simulink model "path_following_revised"  (R2016a)
settings: Solver=ode4  StartTime=0.0  StopTime=2000  FixedStep=0.001  MaxStep=0.01  RelTol=1e-6
values from neighbouring files (symbols this model uses):
  float =     [waveglider.mat]
  floatABC =     [waveglider.mat]
  gliderABC =     [waveglider.mat]
undefined symbols (not defined in the file or in its folder): magnitude, RAO_Vel
libraries: simulink_extras x8, simulink x5, marine_gnc x4, fuzblock x1, marine_hydro x1
(part 3 of 3)

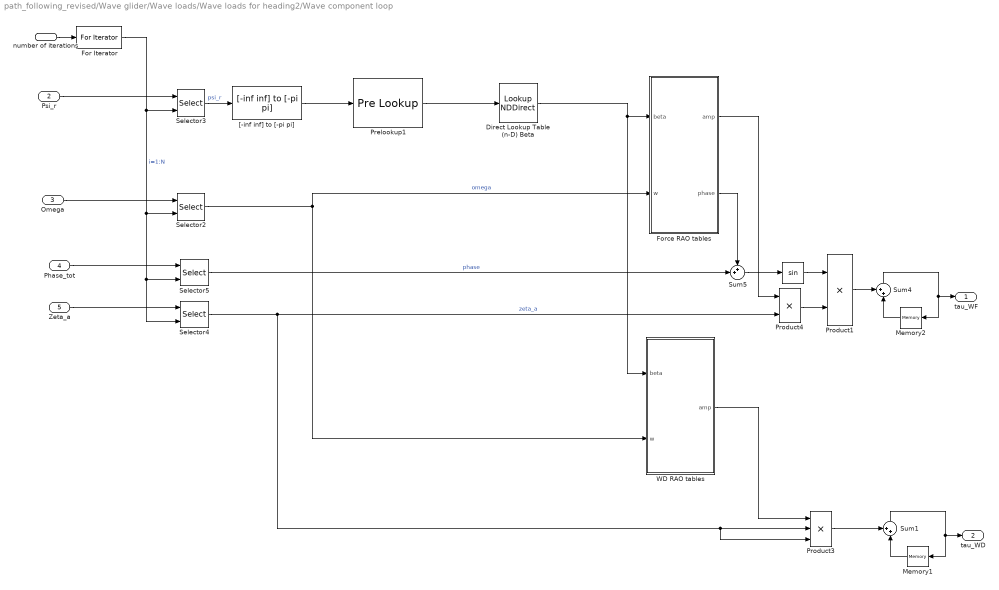
== system path_following_revised/Wave glider/Wave loads/Wave loads for heading2/Wave component loop ==
  number of iterations : Inport
  Psi_r : Inport  Port=2
  Omega : Inport  Port=3
  Phase_tot : Inport  Port=4
  Zeta_a : Inport  Port=5
  "                " : Trigonometry
  Direct Lookup Table (n-D) Beta : LookupNDDirect  NumberOfTableDimensions=1  Table=float.headings
  For Iterator : ForIterator  ResetStates=reset  IterationSource=external  IterationVariableDataType=double
  Force RAO tables : Subsystem  mask(RAO table lookup){}
      mask help:
      | Perform 3D table lookup in 6DOF RAO amplitudes and phases, using the relative wave heading psi_r, wave frequency omega and vessel velocity vel as inputs. See documentation of the Motion RAO block or Force RAO block for details. A warning is issued if the input is outside the range spanned by the RAOs.
      |
      | Author: Oyvind N. Smogeli and Thor I. Fossen, 2005-05-03
  Memory1 : Memory  X0=[0 0 0 0 0 0]'  InheritSampleTime=on
  Memory2 : Memory  X0=[0 0 0 0 0 0]'  InheritSampleTime=on
  Prelookup1 : PreLookup  BreakpointsData=float.headings  IndexSearchMethod=Linear search  BeginIndexSearchUsingPreviousIndexResult=on  OutputOnlyTheIndex=on
  Product1 : Product  SaturateOnIntegerOverflow=on  OutDataTypeStr=Inherit: Same as first input
  Product3 : Product  Inputs=3  SaturateOnIntegerOverflow=on  OutDataTypeStr=Inherit: Same as first input
  Product4 : Product  SaturateOnIntegerOverflow=on  OutDataTypeStr=Inherit: Same as first input
  Selector{2..5} (4 alike) : Selector  IndexOptions=Index vector (port)  Indices=[1 3]  OutputSizes=1
  Sum1 : Sum  Inputs=++|  SaturateOnIntegerOverflow=on
  Sum4 : Sum  Inputs=++|  SaturateOnIntegerOverflow=on
  Sum5 : Sum  Inputs=++|  SaturateOnIntegerOverflow=on
  WD RAO tables : Subsystem  mask(RAO table lookup){}
      mask help:
      | Perform 3D table lookup in 6DOF RAO amplitudes and phases, using the relative wave heading psi_r, wave frequency omega and vessel velocity vel as inputs. See documentation of the Motion RAO block or Force RAO block for details. A warning is issued if the input is outside the range spanned by the RAOs.
      |
      | Author: Oyvind N. Smogeli and Thor I. Fossen, 2005-05-03
  "[-inf inf] to [-pi pi]" : marine_gnc/Utilities/Math Operations/[-inf inf] to [-pi pi]
  tau_WF : Outport
  tau_WD : Outport  Port=2
  wires:
  WD RAO tables/1(amp) -> Product3/1
  Force RAO tables/1(amp) -> Product4/1
  Force RAO tables/2(phase) -> Sum5/1
  Direct Lookup Table (n-D) Beta/1 -> WD RAO tables/1(beta), Force RAO tables/1(beta)
  Prelookup1/1 -> Direct Lookup Table (n-D) Beta/1
  For Iterator/1 -> Selector5/2, Selector4/2, Selector2/2, Selector3/2  "i=1:N"
  Selector2/1 -> WD RAO tables/2(w), Force RAO tables/2(w)  "omega"
  "[-inf inf] to [-pi pi]"/1 -> Prelookup1/1
  Product3/1 -> Sum1/1
  Memory1/1 -> Sum1/2
  Sum1/1 -> tau_WD/1, Memory1/1
  Product4/1 -> Product1/2
  "                "/1 -> Product1/1
  Selector3/1 -> "[-inf inf] to [-pi pi]"/1  "psi_r"
  Selector5/1 -> Sum5/2  "phase"
  Product1/1 -> Sum4/1
  Memory2/1 -> Sum4/2
  Sum4/1 -> tau_WF/1, Memory2/1
  number of iterations/1 -> For Iterator/1
  Omega/1 -> Selector2/1
  Psi_r/1 -> Selector3/1
  Phase_tot/1 -> Selector5/1
  Zeta_a/1 -> Selector4/1
  Sum5/1 -> "                "/1
  Selector4/1 -> Product3/3, Product3/2, Product4/2  "zeta_a"

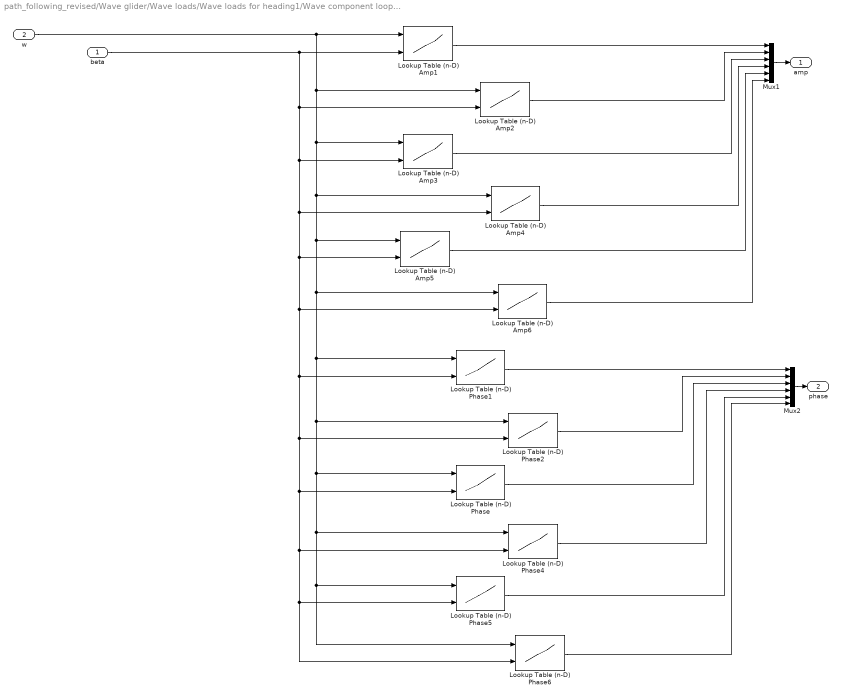
== system path_following_revised/Wave glider/Wave loads/Wave loads for heading1/Wave component loop/Force RAO tables ==
  beta : Inport
  w : Inport  Port=2
  Lookup Table (n-D) Amp1 : Lookup_n-D  BreakpointsForDimension1=float.forceRAO.w  BreakpointsForDimension2=float.headings  BreakpointsForDimension3=RAO_Vel  IndexSearchMethod=Linear search  BeginIndexSearchUsingPreviousIndexResult=on  Table=float.forceRAO.amp{1}  ExtrapMethod=Clip  DiagnosticForOutOfRangeInput=Warning  InternalRulePriority=Speed  RndMeth=Simplest  InputSameDT=on
  Lookup Table (n-D) Amp2 : Lookup_n-D  BreakpointsForDimension1=float.forceRAO.w  BreakpointsForDimension2=float.headings  BreakpointsForDimension3=RAO_Vel  IndexSearchMethod=Linear search  BeginIndexSearchUsingPreviousIndexResult=on  Table=float.forceRAO.amp{2}  ExtrapMethod=Clip  DiagnosticForOutOfRangeInput=Warning  InternalRulePriority=Speed  RndMeth=Simplest  InputSameDT=on
  Lookup Table (n-D) Amp3 : Lookup_n-D  BreakpointsForDimension1=float.forceRAO.w  BreakpointsForDimension2=float.headings  BreakpointsForDimension3=RAO_Vel  IndexSearchMethod=Linear search  BeginIndexSearchUsingPreviousIndexResult=on  Table=float.forceRAO.amp{3}  ExtrapMethod=Clip  DiagnosticForOutOfRangeInput=Warning  InternalRulePriority=Speed  RndMeth=Simplest  InputSameDT=on
  Lookup Table (n-D) Amp4 : Lookup_n-D  BreakpointsForDimension1=float.forceRAO.w  BreakpointsForDimension2=float.headings  BreakpointsForDimension3=RAO_Vel  IndexSearchMethod=Linear search  BeginIndexSearchUsingPreviousIndexResult=on  Table=float.forceRAO.amp{4}  ExtrapMethod=Clip  DiagnosticForOutOfRangeInput=Warning  InternalRulePriority=Speed  RndMeth=Simplest  InputSameDT=on
  Lookup Table (n-D) Amp5 : Lookup_n-D  BreakpointsForDimension1=float.forceRAO.w  BreakpointsForDimension2=float.headings  BreakpointsForDimension3=RAO_Vel  IndexSearchMethod=Linear search  BeginIndexSearchUsingPreviousIndexResult=on  Table=float.forceRAO.amp{5}  ExtrapMethod=Clip  DiagnosticForOutOfRangeInput=Warning  InternalRulePriority=Speed  RndMeth=Simplest  InputSameDT=on
  Lookup Table (n-D) Amp6 : Lookup_n-D  BreakpointsForDimension1=float.forceRAO.w  BreakpointsForDimension2=float.headings  BreakpointsForDimension3=RAO_Vel  IndexSearchMethod=Linear search  BeginIndexSearchUsingPreviousIndexResult=on  Table=float.forceRAO.amp{6}  ExtrapMethod=Clip  DiagnosticForOutOfRangeInput=Warning  InternalRulePriority=Speed  RndMeth=Simplest  InputSameDT=on
  Lookup Table (n-D) Phase : Lookup_n-D  BreakpointsForDimension1=float.forceRAO.w  BreakpointsForDimension2=float.headings  BreakpointsForDimension3=RAO_Vel  IndexSearchMethod=Linear search  BeginIndexSearchUsingPreviousIndexResult=on  Table=float.forceRAO.phase{3}  ExtrapMethod=Clip  DiagnosticForOutOfRangeInput=Warning  InternalRulePriority=Speed  RndMeth=Simplest  InputSameDT=on
  Lookup Table (n-D) Phase1 : Lookup_n-D  BreakpointsForDimension1=float.forceRAO.w  BreakpointsForDimension2=float.headings  BreakpointsForDimension3=RAO_Vel  IndexSearchMethod=Linear search  BeginIndexSearchUsingPreviousIndexResult=on  Table=float.forceRAO.phase{1}  ExtrapMethod=Clip  DiagnosticForOutOfRangeInput=Warning  InternalRulePriority=Speed  RndMeth=Simplest  InputSameDT=on
  Lookup Table (n-D) Phase2 : Lookup_n-D  BreakpointsForDimension1=float.forceRAO.w  BreakpointsForDimension2=float.headings  BreakpointsForDimension3=RAO_Vel  IndexSearchMethod=Linear search  BeginIndexSearchUsingPreviousIndexResult=on  Table=float.forceRAO.phase{2}  ExtrapMethod=Clip  DiagnosticForOutOfRangeInput=Warning  InternalRulePriority=Speed  RndMeth=Simplest  InputSameDT=on
  Lookup Table (n-D) Phase4 : Lookup_n-D  BreakpointsForDimension1=float.forceRAO.w  BreakpointsForDimension2=float.headings  BreakpointsForDimension3=RAO_Vel  IndexSearchMethod=Linear search  BeginIndexSearchUsingPreviousIndexResult=on  Table=float.forceRAO.phase{4}  ExtrapMethod=Clip  DiagnosticForOutOfRangeInput=Warning  InternalRulePriority=Speed  RndMeth=Simplest  InputSameDT=on
  Lookup Table (n-D) Phase5 : Lookup_n-D  BreakpointsForDimension1=float.forceRAO.w  BreakpointsForDimension2=float.headings  BreakpointsForDimension3=RAO_Vel  IndexSearchMethod=Linear search  BeginIndexSearchUsingPreviousIndexResult=on  Table=float.forceRAO.phase{5}  ExtrapMethod=Clip  DiagnosticForOutOfRangeInput=Warning  InternalRulePriority=Speed  RndMeth=Simplest  InputSameDT=on
  Lookup Table (n-D) Phase6 : Lookup_n-D  BreakpointsForDimension1=float.forceRAO.w  BreakpointsForDimension2=float.headings  BreakpointsForDimension3=RAO_Vel  IndexSearchMethod=Linear search  BeginIndexSearchUsingPreviousIndexResult=on  Table=float.forceRAO.phase{6}  ExtrapMethod=Clip  DiagnosticForOutOfRangeInput=Warning  InternalRulePriority=Speed  RndMeth=Simplest  InputSameDT=on
  Mux1 : Mux  Inputs=6
  Mux2 : Mux  Inputs=6
  amp : Outport
  phase : Outport  Port=2
  wires:
  w/1 -> Lookup Table (n-D) Amp1/1, Lookup Table (n-D) Amp2/1, Lookup Table (n-D) Amp3/1, Lookup Table (n-D) Amp4/1, Lookup Table (n-D) Amp5/1, Lookup Table (n-D) Amp6/1, Lookup Table (n-D) Phase1/1, Lookup Table (n-D) Phase2/1, Lookup Table (n-D) Phase/1, Lookup Table (n-D) Phase4/1, Lookup Table (n-D) Phase6/1, Lookup Table (n-D) Phase5/1
  Lookup Table (n-D) Phase5/1 -> Mux2/5
  Lookup Table (n-D) Phase/1 -> Mux2/3
  Lookup Table (n-D) Phase1/1 -> Mux2/1
  beta/1 -> Lookup Table (n-D) Amp1/2, Lookup Table (n-D) Amp2/2, Lookup Table (n-D) Amp3/2, Lookup Table (n-D) Amp4/2, Lookup Table (n-D) Amp6/2, Lookup Table (n-D) Phase1/2, Lookup Table (n-D) Phase2/2, Lookup Table (n-D) Phase/2, Lookup Table (n-D) Phase4/2, Lookup Table (n-D) Phase6/2, Lookup Table (n-D) Phase5/2, Lookup Table (n-D) Amp5/2
  Lookup Table (n-D) Phase4/1 -> Mux2/4
  Lookup Table (n-D) Phase2/1 -> Mux2/2
  Lookup Table (n-D) Phase6/1 -> Mux2/6
  Lookup Table (n-D) Amp4/1 -> Mux1/4
  Lookup Table (n-D) Amp1/1 -> Mux1/1
  Lookup Table (n-D) Amp3/1 -> Mux1/3
  Lookup Table (n-D) Amp5/1 -> Mux1/5
  Lookup Table (n-D) Amp2/1 -> Mux1/2
  Lookup Table (n-D) Amp6/1 -> Mux1/6
  Mux2/1 -> phase/1
  Mux1/1 -> amp/1

== system path_following_revised/Wave glider/Wave loads/Wave loads for heading1/Wave component loop/WD RAO tables ==
  beta : Inport
  w : Inport  Port=2
  Constant : Constant  Value=0
  Lookup Table (n-D) Wavedrift 1 : Lookup_n-D  BreakpointsForDimension1=float.driftfrc.w  BreakpointsForDimension2=float.headings  BreakpointsForDimension3=RAO_Vel  IndexSearchMethod=Linear search  BeginIndexSearchUsingPreviousIndexResult=on  Table=float.driftfrc.amp{1}  ExtrapMethod=Clip  DiagnosticForOutOfRangeInput=Warning  InternalRulePriority=Speed  RndMeth=Simplest  InputSameDT=on
  Lookup Table (n-D) Wavedrift 2 : Lookup_n-D  BreakpointsForDimension1=float.driftfrc.w  BreakpointsForDimension2=float.headings  BreakpointsForDimension3=RAO_Vel  IndexSearchMethod=Linear search  BeginIndexSearchUsingPreviousIndexResult=on  Table=float.driftfrc.amp{2}  ExtrapMethod=Clip  DiagnosticForOutOfRangeInput=Warning  InternalRulePriority=Speed  RndMeth=Simplest  InputSameDT=on
  Lookup Table (n-D) Wavedrift 3 : Lookup_n-D  BreakpointsForDimension1=float.driftfrc.w  BreakpointsForDimension2=float.headings  BreakpointsForDimension3=RAO_Vel  IndexSearchMethod=Linear search  BeginIndexSearchUsingPreviousIndexResult=on  Table=float.driftfrc.amp{3}  ExtrapMethod=Clip  DiagnosticForOutOfRangeInput=Warning  InternalRulePriority=Speed  RndMeth=Simplest  InputSameDT=on
  Mux1 : Mux  Inputs=6
  amp : Outport
  wires:
  w/1 -> Lookup Table (n-D) Wavedrift 1/1, Lookup Table (n-D) Wavedrift 3/1, Lookup Table (n-D) Wavedrift 2/1
  Constant/1 -> Mux1/5, Mux1/4, Mux1/3
  beta/1 -> Lookup Table (n-D) Wavedrift 1/2, Lookup Table (n-D) Wavedrift 3/2, Lookup Table (n-D) Wavedrift 2/2
  Lookup Table (n-D) Wavedrift 1/1 -> Mux1/1
  Lookup Table (n-D) Wavedrift 2/1 -> Mux1/2
  Lookup Table (n-D) Wavedrift 3/1 -> Mux1/6
  Mux1/1 -> amp/1

== system path_following_revised/Wave glider/Wave loads/Wave loads for heading2/Wave component loop/Force RAO tables ==
  beta : Inport
  w : Inport  Port=2
  Lookup Table (n-D) Amp1 : Lookup_n-D  BreakpointsForDimension1=float.forceRAO.w  BreakpointsForDimension2=float.headings  BreakpointsForDimension3=RAO_Vel  IndexSearchMethod=Linear search  BeginIndexSearchUsingPreviousIndexResult=on  Table=float.forceRAO.amp{1}  ExtrapMethod=Clip  DiagnosticForOutOfRangeInput=Warning  InternalRulePriority=Speed  RndMeth=Simplest  InputSameDT=on
  Lookup Table (n-D) Amp2 : Lookup_n-D  BreakpointsForDimension1=float.forceRAO.w  BreakpointsForDimension2=float.headings  BreakpointsForDimension3=RAO_Vel  IndexSearchMethod=Linear search  BeginIndexSearchUsingPreviousIndexResult=on  Table=float.forceRAO.amp{2}  ExtrapMethod=Clip  DiagnosticForOutOfRangeInput=Warning  InternalRulePriority=Speed  RndMeth=Simplest  InputSameDT=on
  Lookup Table (n-D) Amp3 : Lookup_n-D  BreakpointsForDimension1=float.forceRAO.w  BreakpointsForDimension2=float.headings  BreakpointsForDimension3=RAO_Vel  IndexSearchMethod=Linear search  BeginIndexSearchUsingPreviousIndexResult=on  Table=float.forceRAO.amp{3}  ExtrapMethod=Clip  DiagnosticForOutOfRangeInput=Warning  InternalRulePriority=Speed  RndMeth=Simplest  InputSameDT=on
  Lookup Table (n-D) Amp4 : Lookup_n-D  BreakpointsForDimension1=float.forceRAO.w  BreakpointsForDimension2=float.headings  BreakpointsForDimension3=RAO_Vel  IndexSearchMethod=Linear search  BeginIndexSearchUsingPreviousIndexResult=on  Table=float.forceRAO.amp{4}  ExtrapMethod=Clip  DiagnosticForOutOfRangeInput=Warning  InternalRulePriority=Speed  RndMeth=Simplest  InputSameDT=on
  Lookup Table (n-D) Amp5 : Lookup_n-D  BreakpointsForDimension1=float.forceRAO.w  BreakpointsForDimension2=float.headings  BreakpointsForDimension3=RAO_Vel  IndexSearchMethod=Linear search  BeginIndexSearchUsingPreviousIndexResult=on  Table=float.forceRAO.amp{5}  ExtrapMethod=Clip  DiagnosticForOutOfRangeInput=Warning  InternalRulePriority=Speed  RndMeth=Simplest  InputSameDT=on
  Lookup Table (n-D) Amp6 : Lookup_n-D  BreakpointsForDimension1=float.forceRAO.w  BreakpointsForDimension2=float.headings  BreakpointsForDimension3=RAO_Vel  IndexSearchMethod=Linear search  BeginIndexSearchUsingPreviousIndexResult=on  Table=float.forceRAO.amp{6}  ExtrapMethod=Clip  DiagnosticForOutOfRangeInput=Warning  InternalRulePriority=Speed  RndMeth=Simplest  InputSameDT=on
  Lookup Table (n-D) Phase : Lookup_n-D  BreakpointsForDimension1=float.forceRAO.w  BreakpointsForDimension2=float.headings  BreakpointsForDimension3=RAO_Vel  IndexSearchMethod=Linear search  BeginIndexSearchUsingPreviousIndexResult=on  Table=float.forceRAO.phase{3}  ExtrapMethod=Clip  DiagnosticForOutOfRangeInput=Warning  InternalRulePriority=Speed  RndMeth=Simplest  InputSameDT=on
  Lookup Table (n-D) Phase1 : Lookup_n-D  BreakpointsForDimension1=float.forceRAO.w  BreakpointsForDimension2=float.headings  BreakpointsForDimension3=RAO_Vel  IndexSearchMethod=Linear search  BeginIndexSearchUsingPreviousIndexResult=on  Table=float.forceRAO.phase{1}  ExtrapMethod=Clip  DiagnosticForOutOfRangeInput=Warning  InternalRulePriority=Speed  RndMeth=Simplest  InputSameDT=on
  Lookup Table (n-D) Phase2 : Lookup_n-D  BreakpointsForDimension1=float.forceRAO.w  BreakpointsForDimension2=float.headings  BreakpointsForDimension3=RAO_Vel  IndexSearchMethod=Linear search  BeginIndexSearchUsingPreviousIndexResult=on  Table=float.forceRAO.phase{2}  ExtrapMethod=Clip  DiagnosticForOutOfRangeInput=Warning  InternalRulePriority=Speed  RndMeth=Simplest  InputSameDT=on
  Lookup Table (n-D) Phase4 : Lookup_n-D  BreakpointsForDimension1=float.forceRAO.w  BreakpointsForDimension2=float.headings  BreakpointsForDimension3=RAO_Vel  IndexSearchMethod=Linear search  BeginIndexSearchUsingPreviousIndexResult=on  Table=float.forceRAO.phase{4}  ExtrapMethod=Clip  DiagnosticForOutOfRangeInput=Warning  InternalRulePriority=Speed  RndMeth=Simplest  InputSameDT=on
  Lookup Table (n-D) Phase5 : Lookup_n-D  BreakpointsForDimension1=float.forceRAO.w  BreakpointsForDimension2=float.headings  BreakpointsForDimension3=RAO_Vel  IndexSearchMethod=Linear search  BeginIndexSearchUsingPreviousIndexResult=on  Table=float.forceRAO.phase{5}  ExtrapMethod=Clip  DiagnosticForOutOfRangeInput=Warning  InternalRulePriority=Speed  RndMeth=Simplest  InputSameDT=on
  Lookup Table (n-D) Phase6 : Lookup_n-D  BreakpointsForDimension1=float.forceRAO.w  BreakpointsForDimension2=float.headings  BreakpointsForDimension3=RAO_Vel  IndexSearchMethod=Linear search  BeginIndexSearchUsingPreviousIndexResult=on  Table=float.forceRAO.phase{6}  ExtrapMethod=Clip  DiagnosticForOutOfRangeInput=Warning  InternalRulePriority=Speed  RndMeth=Simplest  InputSameDT=on
  Mux1 : Mux  Inputs=6
  Mux2 : Mux  Inputs=6
  amp : Outport
  phase : Outport  Port=2
  wires:
  w/1 -> Lookup Table (n-D) Amp1/1, Lookup Table (n-D) Amp2/1, Lookup Table (n-D) Amp3/1, Lookup Table (n-D) Amp4/1, Lookup Table (n-D) Amp5/1, Lookup Table (n-D) Amp6/1, Lookup Table (n-D) Phase1/1, Lookup Table (n-D) Phase2/1, Lookup Table (n-D) Phase/1, Lookup Table (n-D) Phase4/1, Lookup Table (n-D) Phase6/1, Lookup Table (n-D) Phase5/1
  Lookup Table (n-D) Phase5/1 -> Mux2/5
  Lookup Table (n-D) Phase/1 -> Mux2/3
  Lookup Table (n-D) Phase1/1 -> Mux2/1
  beta/1 -> Lookup Table (n-D) Amp1/2, Lookup Table (n-D) Amp2/2, Lookup Table (n-D) Amp3/2, Lookup Table (n-D) Amp4/2, Lookup Table (n-D) Amp6/2, Lookup Table (n-D) Phase1/2, Lookup Table (n-D) Phase2/2, Lookup Table (n-D) Phase/2, Lookup Table (n-D) Phase4/2, Lookup Table (n-D) Phase6/2, Lookup Table (n-D) Phase5/2, Lookup Table (n-D) Amp5/2
  Lookup Table (n-D) Phase4/1 -> Mux2/4
  Lookup Table (n-D) Phase2/1 -> Mux2/2
  Lookup Table (n-D) Phase6/1 -> Mux2/6
  Lookup Table (n-D) Amp4/1 -> Mux1/4
  Lookup Table (n-D) Amp1/1 -> Mux1/1
  Lookup Table (n-D) Amp3/1 -> Mux1/3
  Lookup Table (n-D) Amp5/1 -> Mux1/5
  Lookup Table (n-D) Amp2/1 -> Mux1/2
  Lookup Table (n-D) Amp6/1 -> Mux1/6
  Mux2/1 -> phase/1
  Mux1/1 -> amp/1

== system path_following_revised/Wave glider/Wave loads/Wave loads for heading2/Wave component loop/WD RAO tables ==
  beta : Inport
  w : Inport  Port=2
  Constant : Constant  Value=0
  Lookup Table (n-D) Wavedrift 1 : Lookup_n-D  BreakpointsForDimension1=float.driftfrc.w  BreakpointsForDimension2=float.headings  BreakpointsForDimension3=RAO_Vel  IndexSearchMethod=Linear search  BeginIndexSearchUsingPreviousIndexResult=on  Table=float.driftfrc.amp{1}  ExtrapMethod=Clip  DiagnosticForOutOfRangeInput=Warning  InternalRulePriority=Speed  RndMeth=Simplest  InputSameDT=on
  Lookup Table (n-D) Wavedrift 2 : Lookup_n-D  BreakpointsForDimension1=float.driftfrc.w  BreakpointsForDimension2=float.headings  BreakpointsForDimension3=RAO_Vel  IndexSearchMethod=Linear search  BeginIndexSearchUsingPreviousIndexResult=on  Table=float.driftfrc.amp{2}  ExtrapMethod=Clip  DiagnosticForOutOfRangeInput=Warning  InternalRulePriority=Speed  RndMeth=Simplest  InputSameDT=on
  Lookup Table (n-D) Wavedrift 3 : Lookup_n-D  BreakpointsForDimension1=float.driftfrc.w  BreakpointsForDimension2=float.headings  BreakpointsForDimension3=RAO_Vel  IndexSearchMethod=Linear search  BeginIndexSearchUsingPreviousIndexResult=on  Table=float.driftfrc.amp{3}  ExtrapMethod=Clip  DiagnosticForOutOfRangeInput=Warning  InternalRulePriority=Speed  RndMeth=Simplest  InputSameDT=on
  Mux1 : Mux  Inputs=6
  amp : Outport
  wires:
  w/1 -> Lookup Table (n-D) Wavedrift 1/1, Lookup Table (n-D) Wavedrift 3/1, Lookup Table (n-D) Wavedrift 2/1
  Constant/1 -> Mux1/5, Mux1/4, Mux1/3
  beta/1 -> Lookup Table (n-D) Wavedrift 1/2, Lookup Table (n-D) Wavedrift 3/2, Lookup Table (n-D) Wavedrift 2/2
  Lookup Table (n-D) Wavedrift 1/1 -> Mux1/1
  Lookup Table (n-D) Wavedrift 2/1 -> Mux1/2
  Lookup Table (n-D) Wavedrift 3/1 -> Mux1/6
  Mux1/1 -> amp/1

== matlab function path_following_revised/LOS  ==
  data: xt input; phid output; yt input
function phid = p_f(xt, yt)
%#%%路径跟踪算法%%
Pt=[yt,xt];
deta=16;
R=10;
%%points_way
P=[ 10,0
    50,200
    200,400
    400,450
    ];  

%判断当前航迹段%
    d=[0,0,0,0];
    for i=1:1:length(P)
        d(i)=norm(P(i,:)-Pt);
    end
    [a,b]=min(d);%寻找与当前位置最近的点的位置
    if b==1
       A=P(b+1,2)-P(b,2);
       B=P(b,1)-P(b+1,1);
       C=P(b+1,1)*P(b,2)-P(b,1)*P(b+1,2);
       y0=(B*B*yt-A*B*xt-A*C)/(A^2+B^2);
       x0=(-A*B*yt+A^2*xt-B*C)/(A^2+B^2);%求出垂足
       yd=y0-sign(P(b,1)-P(b+1,1))*sqrt((deta^2)/(1+(abs(P(b,2)-P(b+1,2))/(P(b,1)-P(b+1,1)))^2));
       xd=x0-sign(P(b,2)-P(b+1,2))*(abs(P(b,2)-P(b+1,2))/(P(b,1)-P(b+1,1)))*(y0-yd);%求出LOS点
       %%计算期望航向
       e = sqrt((xd-xt)^2+(yd-yt)^2)-R;
        if e>0
            phid=direction(xd, yd, xt, yt);
        else
            phid=direction(P(b+1,2),P(b+1,1),P(b,2),P(b,1));
        end
        
    elseif b==length(P)
       A=P(b,2)-P(b-1,2);
       B=P(b-1,1)-P(b,1);
       C=P(b,1)*P(b-1,2)-P(b-1,1)*P(b,2);
       y0=(B*B*yt-A*B*xt-A*C)/(A^2+B^2);
       x0=(-A*B*yt+A^2*xt-B*C)/(A^2+B^2);%求出垂足;
       yd=y0-sign(P(b-1,1)-P(b,1))*sqrt((deta^2)/(1+(abs(P(b-1,2)-P(b,2))/(P(b-1,1)-P(b,1)))^2));
       xd=x0-sign(P(b-1,2)-P(b,2))*(abs(P(b-1,2)-P(b,2))/(P(b-1,1)-P(b,1)))*(y0-yd);
       %%计算期望航向
       e = sqrt((xd-xt)^2+(yd-yt)^2)-R;
        if e>0
            phid=direction(xd, yd, xt, yt);
        else
            phid=direction(P(b,2),P(b,1),P(b-1,2),P(b-1,1));
        end
    else
        PbPt=Pt-P(b,:);
        PbPb_1=P(b-1,:)-P(b,:);
        PbPb1=P(b+1,:)-P(b,:);
        if angle(PbPt,PbPb_1)<angle(PbPt,PbPb1)
           A=P(b,2)-P(b-1,2);
           B=P(b-1,1)-P(b,1);
           C=P(b,1)*P(b-1,2)-P(b-1,1)*P(b,2);
           y0=(B*B*yt-A*B*xt-A*C)/(A^2+B^2);
           x0=(-A*B*yt+A^2*xt-B*C)/(A^2+B^2);%求出垂足;
           yd=y0-sign(P(b-1,1)-P(b,1))*sqrt((deta^2)/(1+(abs(P(b-1,2)-P(b,2))/(P(b-1,1)-P(b,1)))^2));
           xd=x0-sign(P(b-1,2)-P(b,2))*(abs(P(b-1,2)-P(b,2))/(P(b-1,1)-P(b,1)))*(y0-yd);
              %%计算期望航向
           e = sqrt((xd-xt)^2+(yd-yt)^2)-R;
            if e>0
                phid=direction(xd, yd, xt, yt);
            else
                phid=direction(P(b,2),P(b,1),P(b-1,2),P(b-1,1));
            end
        else
           A=P(b+1,2)-P(b,2);
           B=P(b,1)-P(b+1,1);
           C=P(b+1,1)*P(b,2)-P(b,1)*P(b+1,2);
           y0=(B*B*yt-A*B*xt-A*C)/(A^2+B^2);
           x0=(-A*B*yt+A^2*xt-B*C)/(A^2+B^2);%求出垂足
           yd=y0-sign(P(b,1)-P(b+1,1))*sqrt((deta^2)/(1+(abs(P(b,2)-P(b+1,2))/(P(b,1)-P(b+1,1)))^2));
           xd=x0-sign(P(b,2)-P(b+1,2))*(abs(P(b,2)-P(b+1,2))/(P(b,1)-P(b+1,1)))*(y0-yd);
                  %%计算期望航向
           e = sqrt((xd-xt)^2+(yd-yt)^2)-R;
            if e>0
                phid=direction(xd, yd, xt, yt);
            else
                phid=direction(P(b+1,2),P(b+1,1),P(b,2),P(b,1));
            end
        end
    end

end

== matlab function path_following_revised/Wave glider/Hydrofoil force/steady foilforce/MATLAB Function ==
  data: alpha input; CL output; Cdc input; lamda input; eks input
function CL = fcn(alpha,Cdc,lamda,eks)
%#codegen

CL = 1.8*pi*lamda*alpha/(cos(eks)*sqrt(lamda^2/cos(eks)^4+4)+1.8)+Cdc*alpha^2/lamda;

== matlab function path_following_revised/Wave glider/Rudder/MATLAB Function ==
  data: alpha input; Cl output; Cdc input; lamda input; eks input
function Cl = fcn(alpha,Cdc,lamda,eks)
%#codegen

Cl = 1.8*pi*lamda*alpha/(cos(eks)*sqrt(lamda^2/cos(eks)^4+4)+1.8)+Cdc*alpha^2/lamda;

== matlab function path_following_revised/Wave glider/tether tension/MATLAB Function ==
  data: x input; T output; y input; z input; alpha output; beta output
function [T,alpha,beta] = fcn(x,y,z)
%#codegen
T=1.7e+7*(sqrt(x^2+y^2+z^2)-6.2)+200;
if T<0
    T=0;
end
alpha=0;
if x>0
    alpha=atan(y/x);
elseif x<0
    alpha=atan(y/x)+pi;
elseif x==0
    if y>0
        alpha=pi/2;
    elseif y==0
        alpha=0;
    else alpha=-pi/2;
    end
end
beta=asin(sqrt((x^2+y^2)/(x^2+y^2+z^2)));
